simulink subsystem "OL"  (R2024a)
settings: Solver=VariableStepAuto  StartTime=0.0  StopTime=10.0  RelTol=1e-3
libraries: px4lib x3
settings Model: Creator=gurt1  LastModifiedBy=gurt1

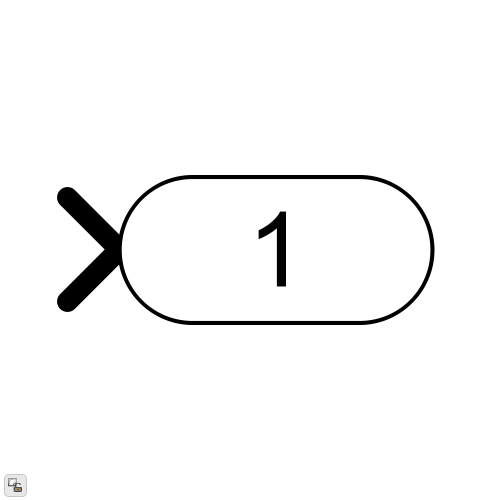
[thumbnail: Simulink's stored preview of the top-level diagram]
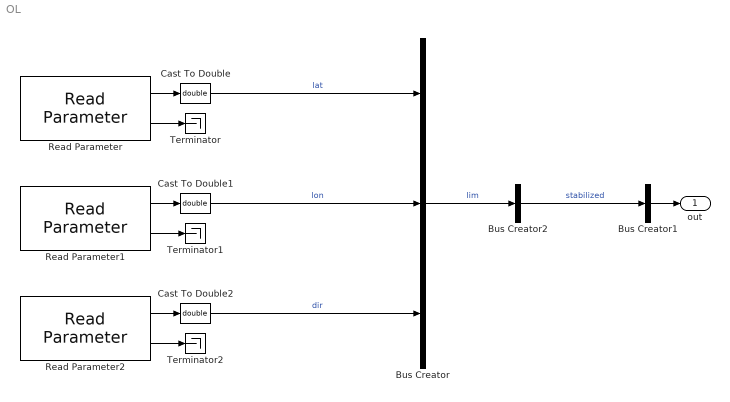
== system OL ==
  Bus Creator : BusCreator  Inputs=3
  Bus Creator1 : BusCreator  Inputs=1
  Bus Creator2 : BusCreator  Inputs=1
  Cast To Double : DataTypeConversion  OutDataTypeStr=double  SaturateOnIntegerOverflow=off  RndMeth=Floor
  Cast To Double1 : DataTypeConversion  OutDataTypeStr=double  SaturateOnIntegerOverflow=off  RndMeth=Floor
  Cast To Double2 : DataTypeConversion  OutDataTypeStr=double  SaturateOnIntegerOverflow=off  RndMeth=Floor
  Read Parameter : px4lib/Read Parameter  ParameterName=OL_STAB_LAT_LIM  DataType=FLOAT  SampleTime=-1
  Read Parameter1 : px4lib/Read Parameter  ParameterName=OL_STAB_LON_LIM  DataType=FLOAT  SampleTime=-1
  Read Parameter2 : px4lib/Read Parameter  ParameterName=OL_STAB_DIR_LIM  DataType=FLOAT  SampleTime=-1
  Terminator : Terminator
  Terminator1 : Terminator
  Terminator2 : Terminator
  out : Outport
  wires:
  Read Parameter/2 -> Terminator/1
  Read Parameter/1 -> Cast To Double/1
  Cast To Double/1 -> Bus Creator/1  "lat"
  Bus Creator1/1 -> out/1
  Bus Creator/1 -> Bus Creator2/1  "lim"
  Bus Creator2/1 -> Bus Creator1/1  "stabilized"
  Read Parameter1/1 -> Cast To Double1/1
  Read Parameter1/2 -> Terminator1/1
  Cast To Double1/1 -> Bus Creator/2  "lon"
  Read Parameter2/2 -> Terminator2/1
  Read Parameter2/1 -> Cast To Double2/1
  Cast To Double2/1 -> Bus Creator/3  "dir"
